simulink model "Final_System_Model_V10"  (R2018a)
settings: Solver=VariableStepAuto  StartTime=0  StopTime=250  FixedStep=0.5  RelTol=1e-3
PreLoadFcn:
  | Ts_Power=1e-6;
  | Ts_Control=100e-6;
undefined symbols (not defined in the file): DiscIntNeverNeededParam, sigbuilder_block
libraries: simulink x24, fl_lib x16, powerlib x15, nesl_utility x8, powerlib_meascontrol x5, re_lib x1
(part 4 of 8)

== system Final_System_Model_V10/Full System/Subsystem1/100KW Fuel Cell Stack_2/Load ==
  note: This Block models the Load Profile as dictated by the ship Resistance in the River Nile
  Signal : Inport
  Bus Selector : BusSelector  OutputSignals=Cell Output Voltage (V),Number Of Cells
  Current from Load profile of one day : Subsystem  Tag=STV Subsys  LoadFcn=sigbuilder_block('load');  StartFcn=sigbuilder_block('start');  StopFcn=sigbuilder_block('stop');  ClipboardFcn=sigbuilder_block('clipboard');  mask(Sigbuilder block){tuvar=[0:10]}
      mask help: Simulink:masks:SigbuilderBlock_MD
      mask init:
      | if ~strcmp(get_param(bdroot(gcbh),'SimulationStatus'),'stopped') tuvar = sigbuilder_block('maskInit'); end
      settings: CopyFcn=sigbuilder_block('copy');  DeleteFcn=sigbuilder_block('delete');  ModelCloseFcn=sigbuilder_block('modelClose');  PreSaveFcn=sigbuilder_block('preSave');  PauseFcn=sigbuilder_block('pause');  ContinueFcn=sigbuilder_block('continue');  NameChangeFcn=sigbuilder_block('namechange');  OpenFcn=sigbuilder_block('open',[403.5 117 550.5 359.25 ]);  CloseFcn=sigbuilder_block('close');
      mask Display: plot(0, 0, 100, 100,[2, 2, 32, 32, 2], [68, 8, 8, 68, 68],[32, 2], [38, 38], [32, 19, 2],[53, 60, 44], [32, 17, 17, 2],[16, 16, 31, 31]);txt = getActiveGroup(gcbh);text(2, 100, txt,'verticalAlignment', 'top');
  Product : Product
  Terminator : Terminator
  Terminator1 : Terminator
  Total Output Voltage (V) : Outport
  wires:
  Signal/1 -> Bus Selector/1
  Bus Selector/1 -> Product/1  "<Cell Output Voltage (V)>"
  Product/1 -> Total Output Voltage (V)/1  "Total Output Voltage (V)"
  Current from Load profile of one day/2(Signal 2) -> Terminator1/1  "Current from Load profile (Alex to Aswan)"
  Bus Selector/2 -> Product/2  "<Number Of Cells>"
  Current from Load profile of one day/1(Signal 1) -> Terminator/1  "Current from Load profile (Alex to Aswan)"

== system Final_System_Model_V10/Full System/Subsystem1/80KW Fuel Cell Stack_1/From Load Current and Fuel Cell Output Current (A) to Valve Restriction Area (m^2) ==
  note: This block is the feedback block that controls the Flow control valve of the Hydrogen feeding system
      | I NPUTS: A) load Current (A) OUTPUTS: A) valve Restriction Area(m^2) as dictated by the Load Current
      | B) Output Current of the Fuel Cell (A) B) valve Restriction Area (m^2) as dictated by the Fuel Cell output current
  note: FEEDBACK BLOCK
  note: (3.0735e-14*(u(1)^3)) + (-5.0428e-11*(u(1)^2)) +(4.1772e-08*u(1)) + 2.7105e-07
  Load Profile Current (A) : Inport
  Output Current : Inport  Port=2
  Constant1 : Constant  Value=2.016e-3
  Constant2 : Constant  Value=96485
  Constant3 : Constant  Value=2
  Divide : Product  Inputs=*/
  Number Of Cells : Constant  Value=208
  Product : Product  Inputs=3
  Product1 : Product
  Subsystem : Subsystem
  Subsystem1 : Subsystem
  Valve Opening : Outport
  Valve Opening from Output Current : Outport  Port=2
  Hydrogen Mass Flow Rate (Kg/s) : Outport  Port=3
  wires:
  Divide/1 -> Hydrogen Mass Flow Rate (Kg/s)/1
  Constant2/1 -> Product1/1
  Constant3/1 -> Product1/2
  Product1/1 -> Divide/2
  Constant1/1 -> Product/3
  Number Of Cells/1 -> Product/2
  Product/1 -> Divide/1
  Subsystem1/1(Out1) -> Valve Opening/1
  Load Profile Current (A)/1 -> Subsystem1/1(In1)
  Subsystem/1(Valve Opening from Output Current) -> Valve Opening from Output Current/1
  Output Current/1 -> Subsystem/1(In1), Product/1

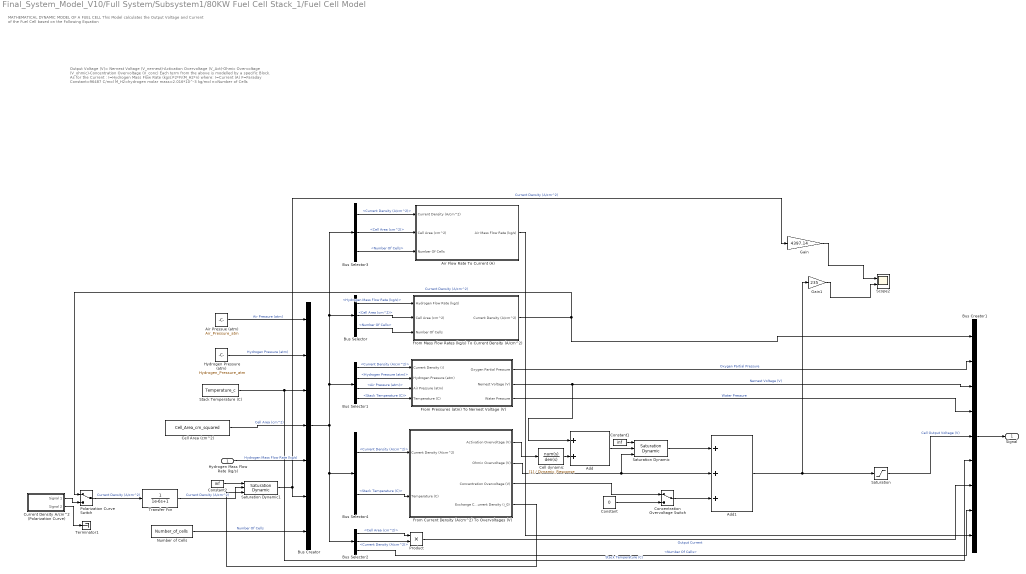
== system Final_System_Model_V10/Full System/Subsystem1/80KW Fuel Cell Stack_1/Fuel Cell Model ==
  note: MATHEMATICAL DYNAMIC MODEL OF A FUEL CELL
      | This Model calculates the Output Voltage and Current of the Fuel Cell based on the Following Equation
  note: Output Voltage (V)= Nernest Voltage (V_nernest)-Activation Overvoltage (V_Act)-Ohmic Overvoltage (V_ohmic)-Concentration Overvoltage (V_conc)
      | Each term from the above is modelled by a specific Block.
      | As for the Current :
      |
      | I=Hydrogen Mass Flow Rate (kg/s)*2*F/(M_H2*n)
      | where: I=Current (A)
      | F=Faraday Constant=96487 C/mol
      | M_H2=hydrogen molar mass=2.016*10^-3 kg/mol
      | n=Number of Cells
  Hydrogen Mass Flow Rate (kg/s) : Inport
  " From Current Density (A/cm^2) To Overvoltages (V)" : Subsystem
  Add : Sum
  Add1 : Sum  Inputs=+++
  Air Flow Rate To Current (A) : Subsystem
  Air Pressue (atm) : Constant  Value=Air_Pressure_atm
  Bus Creator : BusCreator  Inputs=7
  Bus Creator1 : BusCreator  Inputs=9
  Bus Selector : BusSelector  OutputSignals=Hydrogen Mass Flow Rate (kg/s),Cell Area (cm^2),Number Of Cells
  Bus Selector1 : BusSelector  OutputSignals=Current Density (A/cm^2),Hydrogen Pressure (atm),Air Pressure (atm),Stack Temperature (C)
  Bus Selector2 : BusSelector  OutputSignals=Cell Area (cm^2),Current Density (A/cm^2),Number Of Cells
  Bus Selector3 : BusSelector  OutputSignals=Current Density (A/cm^2),Cell Area (cm^2),Number Of Cells
  Bus Selector4 : BusSelector  OutputSignals=Current Density (A/cm^2),Stack Temperature (C)
  Cell Area (cm^2) : Constant  Value=Cell_Area_cm_squared
  Cell dynamic : TransferFcn  Denominator=Dynamic_Response
  Concentration Overvoltage Switch : ManualSwitch
  Constant : Constant  Value=0
  Constant1 : Constant  Value=inf
  Constant2 : Constant  Value=inf
  Current Density A/cm^2 (Polarization Curve) : Subsystem  Tag=STV Subsys  LoadFcn=sigbuilder_block('load');  StartFcn=sigbuilder_block('start');  StopFcn=sigbuilder_block('stop');  ClipboardFcn=sigbuilder_block('clipboard');  mask(Sigbuilder block){tuvar=[0:10]}
      mask help: Simulink:masks:SigbuilderBlock_MD
      mask init:
      | if ~strcmp(get_param(bdroot(gcbh),'SimulationStatus'),'stopped') tuvar = sigbuilder_block('maskInit'); end
      settings: CopyFcn=sigbuilder_block('copy');  DeleteFcn=sigbuilder_block('delete');  ModelCloseFcn=sigbuilder_block('modelClose');  PreSaveFcn=sigbuilder_block('preSave');  PauseFcn=sigbuilder_block('pause');  ContinueFcn=sigbuilder_block('continue');  NameChangeFcn=sigbuilder_block('namechange');  OpenFcn=sigbuilder_block('open',[403.5 117 550.5 359.25 ]);  CloseFcn=sigbuilder_block('close');
      mask Display: plot(0, 0, 100, 100,[2, 2, 32, 32, 2], [68, 8, 8, 68, 68],[32, 2], [38, 38], [32, 19, 2],[53, 60, 44], [32, 17, 17, 2],[16, 16, 31, 31]);txt = getActiveGroup(gcbh);text(2, 100, txt,'verticalAlignment', 'top');
  From Mass Flow Rates (kg/s) To Current Density (A/cm^2) : Subsystem
  From Pressures (atm) To Nernest Voltage (V) : Subsystem
  Gain : Gain  Gain=4397.14
  Gain1 : Gain  Gain=235
  Hydrogen Pressure (atm) : Constant  Value=Hydrogen_Pressure_atm
  Number of Cells : Constant  Value=Number_of_cells
  Polarization Curve Switch : ManualSwitch
  Product : Product
  Saturation : Saturate  UpperLimit=inf  LowerLimit=0  ZeroCross=off
  Saturation Dynamic : simulink/Discontinuities/Saturation Dynamic  OutMin=[]  OutMax=[]  OutDataTypeStr=Inherit: Same as second input  OutDataType=sfix(16)  OutScaling=2^-10  DoSatur=off
  Saturation Dynamic1 : simulink/Discontinuities/Saturation Dynamic  OutMin=[]  OutMax=[]  OutDataTypeStr=Inherit: Same as second input  OutDataType=sfix(16)  OutScaling=2^-10  DoSatur=off
  Scope2 : Scope  NumInputPorts=2
  Stack Temperature (C) : Constant  Value=Temperature_c
  Terminator1 : Terminator
  Transfer Fcn : TransferFcn  Denominator=[1e-6 1]
  Signal : Outport
  wires:
  Bus Selector3/3 -> Air Flow Rate To Current (A)/3(Number Of Cells)  "<Number Of Cells>"
  Bus Selector3/2 -> Air Flow Rate To Current (A)/2(Cell Area (cm^2))  "<Cell Area (cm^2)>"
  Bus Selector3/1 -> Air Flow Rate To Current (A)/1(Current Density (A/cm^2))  "<Current Density (A/cm^2)>"
  Gain1/1 -> Scope2/2
  Gain/1 -> Scope2/1
  Current Density A/cm^2 (Polarization Curve)/2(Signal 2) -> Terminator1/1
  Air Flow Rate To Current (A)/1(Air Mass Flow Rate (kg/s)) -> Bus Creator1/9
  Constant/1 -> Concentration Overvoltage Switch/2
  Concentration Overvoltage Switch/1 -> Add1/3
  " From Current Density (A/cm^2) To Overvoltages (V)"/2(Ohmic Overvoltage (V)) -> Add1/2, Saturation Dynamic/3
  Cell Area (cm^2)/1 -> Bus Creator/4  "Cell Area (cm^2)"
  Number of Cells/1 -> Bus Creator/7  "Number Of Cells"
  Air Pressue (atm)/1 -> Bus Creator/1  "Air Pressure (atm)"
  Hydrogen Pressure (atm)/1 -> Bus Creator/2  "Hydrogen Pressure (atm)"
  Stack Temperature (C)/1 -> Bus Creator1/6, Bus Creator/3  "Stack Temperature (C)"
  Transfer Fcn/1 -> Saturation Dynamic1/2  "Current Density (A/cm^2)"
  Saturation Dynamic1/1 -> Gain/1, Bus Creator/6  "Current Density (A/cm^2)"
  Bus Selector2/3 -> Bus Creator1/8  "<Number Of Cells>"
  Bus Selector/3 -> From Mass Flow Rates (kg/s) To Current Density (A/cm^2)/3(Number Of Cells)  "<Number Of Cells>"
  Product/1 -> Bus Creator1/7  "Output Current"
  Bus Selector2/1 -> Product/1  "<Cell Area (cm^2)>"
  Bus Selector2/2 -> Product/2  "<Current Density (A/cm^2)>"
  " From Current Density (A/cm^2) To Overvoltages (V)"/3(Concentration Overvoltage (V)) -> Concentration Overvoltage Switch/1
  Saturation Dynamic/1 -> Add1/1
  Constant1/1 -> Saturation Dynamic/1
  Add/1 -> Saturation Dynamic/2
  Cell dynamic/1 -> Add/2
  Add1/1 -> Saturation/1, Gain1/1
  " From Current Density (A/cm^2) To Overvoltages (V)"/4(Exchange Current Density (i_0)) -> Saturation Dynamic1/3
  Constant2/1 -> Saturation Dynamic1/1
  Polarization Curve Switch/1 -> Transfer Fcn/1  "Current Density (A/cm^2)"
  Bus Creator1/1 -> Signal/1
  " From Current Density (A/cm^2) To Overvoltages (V)"/1(Activation Overvoltage (V)) -> Cell dynamic/1
  Bus Selector4/2 -> " From Current Density (A/cm^2) To Overvoltages (V)"/2(Temperature (C))  "<Stack Temperature (C)>"
  Bus Selector4/1 -> " From Current Density (A/cm^2) To Overvoltages (V)"/1(Current Density (A/cm^2))  "<Current Density (A/cm^2)>"
  From Pressures (atm) To Nernest Voltage (V)/3(Water Pressure) -> Bus Creator1/4  "Water Pressure"
  From Pressures (atm) To Nernest Voltage (V)/1(Oxygen Partial Pressure) -> Bus Creator1/2  "Oxygen Partial Pressure"
  Bus Selector1/4 -> From Pressures (atm) To Nernest Voltage (V)/4(Temperature (C))  "<Stack Temperature (C)>"
  Bus Selector1/3 -> From Pressures (atm) To Nernest Voltage (V)/3(Air Pressure (atm))  "<Air Pressure (atm)>"
  Bus Selector1/2 -> From Pressures (atm) To Nernest Voltage (V)/2(Hydrogen Pressure (atm))  "<Hydrogen Pressure (atm)>"
  Bus Selector1/1 -> From Pressures (atm) To Nernest Voltage (V)/1(Current Density (i))  "<Current Density (A/cm^2)>"
  From Pressures (atm) To Nernest Voltage (V)/2(Nernest Voltage (V)) -> Add/1, Bus Creator1/3  "Nernest Voltage (V)"
  Bus Selector/2 -> From Mass Flow Rates (kg/s) To Current Density (A/cm^2)/2(Cell Area (cm^2))  "<Cell Area (cm^2)>"
  Bus Selector/1 -> From Mass Flow Rates (kg/s) To Current Density (A/cm^2)/1(Hydrogen Flow Rate (kg/s))  "<Hydrogen Mass Flow Rate (kg/s)>"
  From Mass Flow Rates (kg/s) To Current Density (A/cm^2)/1(Current Density (A/cm^2)) -> Polarization Curve Switch/1, Bus Creator1/1  "Current Density (A/cm^2)"
  Bus Creator/1 -> Bus Selector/1, Bus Selector3/1, Bus Selector1/1, Bus Selector4/1, Bus Selector2/1
  Hydrogen Mass Flow Rate (kg/s)/1 -> Bus Creator/5  "Hydrogen Mass Flow Rate (kg/s)"
  Current Density A/cm^2 (Polarization Curve)/1(Signal 1) -> Polarization Curve Switch/2
  Saturation/1 -> Bus Creator1/5  "Cell Output Voltage (V)"
